simulink model "dyn_model"  (R2019a)
settings: Solver=VariableStepAuto  StartTime=0.0  StopTime=40  RelTol=1e-3
values from neighbouring files (symbols this model uses):
  Detal_ref = zeros(N,1)    [path_generate.m]
  Phi_dot_ref = zeros(N,1)    [path_generate.m]
  Phi_ref = phi_ref    [path_generate.m]
  X_dot_ref = zeros(N,1)    [path_generate.m]
  X_ref = X_phi'    [path_generate.m]
  Y_dot_ref = zeros(N,1)    [path_generate.m]
  Y_ref = zeros(N,1)    [path_generate.m]
libraries: Solver_SF x1
settings Model: Creator=Administrator  LastModifiedBy=Administrator

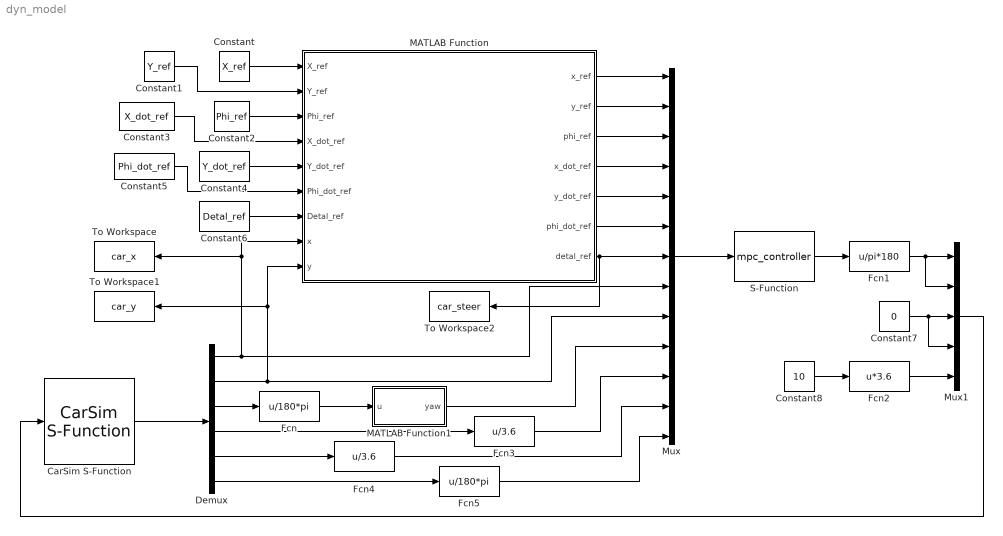
== system dyn_model ==
  CarSim S-Function : Solver_SF/CarSim S-Function  Priority=1  SIMFILE=simfile.sim  Run_RTs=off  vs_state_ind=Run  StopMode_ind=Vehicle Model
  Constant : Constant  Value=X_ref
  Constant1 : Constant  Value=Y_ref
  Constant2 : Constant  Value=Phi_ref
  Constant3 : Constant  Value=X_dot_ref
  Constant4 : Constant  Value=Y_dot_ref
  Constant5 : Constant  Value=Phi_dot_ref
  Constant6 : Constant  Value=Detal_ref
  Constant7 : Constant  Value=0
  Constant8 : Constant  Value=10
  Demux : Demux  Outputs=6
  Fcn : Fcn  Expr=u/180*pi
  Fcn1 : Fcn  Expr=u/pi*180
  Fcn2 : Fcn  Expr=u*3.6
  Fcn3 : Fcn  Expr=u/3.6
  Fcn4 : Fcn  Expr=u/3.6
  Fcn5 : Fcn  Expr=u/180*pi
  MATLAB Function : MATLAB Function  TreatAsAtomicUnit=on
  MATLAB Function1 : MATLAB Function  TreatAsAtomicUnit=on
  Mux : Mux  Inputs=13
  Mux1 : Mux  Inputs=5
  S-Function : S-Function  FunctionName=mpc_controller  SFunctionDeploymentMode=off  EnableBusSupport=off
  To Workspace : ToWorkspace  VariableName=car_x  SampleTime=0.1
      settings: Save2DSignal=2-D array (concatenate along first dimension)
  To Workspace1 : ToWorkspace  VariableName=car_y  SampleTime=0.1
      settings: Save2DSignal=2-D array (concatenate along first dimension)
  To Workspace2 : ToWorkspace  VariableName=car_steer  SampleTime=0.1
      settings: Save2DSignal=2-D array (concatenate along first dimension)
  wires:
  Constant/1 -> MATLAB Function/1(X_ref)
  Constant1/1 -> MATLAB Function/2(Y_ref)
  Constant2/1 -> MATLAB Function/3(Phi_ref)
  Constant3/1 -> MATLAB Function/4(X_dot_ref)
  Constant4/1 -> MATLAB Function/5(Y_dot_ref)
  Constant5/1 -> MATLAB Function/6(Phi_dot_ref)
  Constant6/1 -> MATLAB Function/7(Detal_ref)
  MATLAB Function/5(y_dot_ref) -> Mux/5
  MATLAB Function/1(x_ref) -> Mux/1
  MATLAB Function/2(y_ref) -> Mux/2
  MATLAB Function/3(phi_ref) -> Mux/3
  MATLAB Function/4(x_dot_ref) -> Mux/4
  MATLAB Function/6(phi_dot_ref) -> Mux/6
  MATLAB Function/7(detal_ref) -> To Workspace2/1, Mux/7
  Mux/1 -> S-Function/1
  CarSim S-Function/1 -> Demux/1
  Demux/1 -> MATLAB Function/8(x), To Workspace/1, Mux/8
  Demux/2 -> MATLAB Function/9(y), To Workspace1/1, Mux/9
  Demux/4 -> Fcn3/1
  Demux/5 -> Fcn4/1
  Demux/6 -> Fcn5/1
  Demux/3 -> Fcn/1
  Fcn/1 -> MATLAB Function1/1(u)
  MATLAB Function1/1(yaw) -> Mux/10
  Constant7/1 -> Mux1/3, Mux1/4
  Fcn1/1 -> Mux1/1, Mux1/2
  S-Function/1 -> Fcn1/1
  Constant8/1 -> Fcn2/1
  Fcn2/1 -> Mux1/5
  Mux1/1 -> CarSim S-Function/1
  Fcn3/1 -> Mux/11
  Fcn4/1 -> Mux/12
  Fcn5/1 -> Mux/13

== matlab function dyn_model/MATLAB Function1 ==
  data: u input; yaw output
function yaw = angle_norm(u)
while u<-2*pi
    u=u+2*pi;
end
while u>2*pi
    u=u-2*pi;
end
yaw = u;

== matlab function dyn_model/MATLAB Function ==
  data: X_ref input; x_ref output; y_ref output; phi_ref output; x_dot_ref output; y_dot_ref output; phi_dot_ref output; detal_ref output; Y_ref input; Phi_ref input; X_dot_ref input; Y_dot_ref input; Phi_dot_ref input; Detal_ref input; x input; y input
function [x_ref,y_ref,phi_ref,x_dot_ref,y_dot_ref,phi_dot_ref,detal_ref]...
    = get_ref_data(X_ref,Y_ref,Phi_ref,X_dot_ref,Y_dot_ref,Phi_dot_ref,Detal_ref,x,y)
    N=size(X_ref,1);
    min_dis=99999;
    index=1;
    for i=1:N
        cur_dis=sqrt( (x-X_ref(i))^2+(y-Y_ref(i))^2 );
        if cur_dis<min_dis
            index=i;
            min_dis=cur_dis;
        end
    end
    [x_ref,y_ref,phi_ref]=deal(X_ref(index),Y_ref(index),Phi_ref(index));
    [x_dot_ref,y_dot_ref,phi_dot_ref]=deal(X_dot_ref(index),Y_dot_ref(index),Phi_dot_ref(index));
    detal_ref=Detal_ref(index);
